simulink model "DCmotor"  (R2021a)
settings: Solver=FixedStepAuto  StartTime=0.0  StopTime=0.4  FixedStep=0.0002  RelTol=1e-3
values from neighbouring files (symbols this model uses):
  c_ss = 0.7    [Parametry_SS_motoru.m]    (also in SimRun.m = meas.c_ss + delta(5))
  J = 0.08    [Parametry_SS_motoru.m]    (also in SimRun.m = meas.J + delta(7))
  L_a = 0.8    [Parametry_SS_motoru.m]    (also in SimRun.m = meas.L_a + delta(3))
  L_b = 9.7    [Parametry_SS_motoru.m]    (also in SimRun.m = meas.L_b + delta(4))
  M_z = 0    [Parametry_SS_motoru.m]    (also in SimRun.m = meas.M_z + delta(6))
  R_a = 2.8    [Parametry_SS_motoru.m]    (also in SimRun.m = meas.R_a + delta(1))
  R_b = 8    [Parametry_SS_motoru.m]    (also in SimRun.m = meas.R_b + delta(2))
  U_a = 60.8    [Mereni.m]    (also in Optim.m = 120; Parametry_SS_motoru.m = 100; SimRun.m = U_a + delta(8))
  U_b = 27.6    [Mereni.m]    (also in Optim.m = 120; Parametry_SS_motoru.m = 120; SimRun.m = U_b + delta(9))
settings Model: Creator=liesk  LastModifiedBy=vojta
settings SolverCC: AlgebraicLoopSolver=TrustRegion
settings DebuggingCC: SFMachineParentedDataDiag=warning

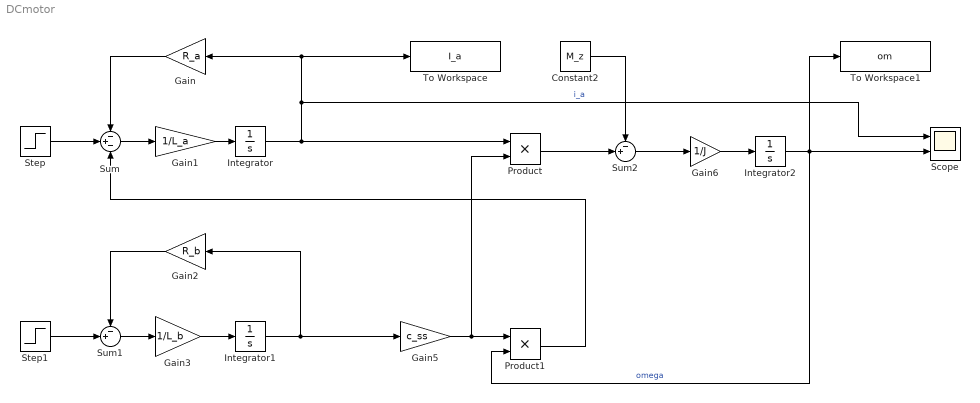
== system DCmotor ==
  Constant2 : Constant  Value=M_z
  Gain : Gain  Gain=R_a
  Gain1 : Gain  Gain=1/L_a
  Gain2 : Gain  Gain=R_b
  Gain3 : Gain  Gain=1/L_b
  Gain5 : Gain  Gain=c_ss
  Gain6 : Gain  Gain=1/J
  Integrator : Integrator
  Integrator1 : Integrator
  Integrator2 : Integrator
  Product : Product
  Product1 : Product
  Scope : Scope  NumInputPorts=2
  Step : Step  Time=0  After=U_a  SampleTime=0
  Step1 : Step  Time=0  After=U_b  SampleTime=0
  Sum : Sum  Inputs=-+-
  Sum1 : Sum  Inputs=-+|
  Sum2 : Sum  Inputs=-+|
  To Workspace : ToWorkspace  VariableName=I_a  SaveFormat=Timeseries  SampleTime=-1
  To Workspace1 : ToWorkspace  VariableName=om  SaveFormat=Timeseries  SampleTime=-1
  wires:
  Gain/1 -> Sum/1
  Sum/1 -> Gain1/1
  Gain1/1 -> Integrator/1
  Integrator/1 -> Gain/1, To Workspace/1, Scope/1, Product/1  "i_a"
  Sum1/1 -> Gain3/1
  Gain3/1 -> Integrator1/1
  Gain2/1 -> Sum1/1
  Step/1 -> Sum/2
  Step1/1 -> Sum1/2
  Product1/1 -> Sum/3
  Integrator1/1 -> Gain5/1, Gain2/1
  Gain5/1 -> Product/2, Product1/1
  Constant2/1 -> Sum2/1
  Product/1 -> Sum2/2
  Gain6/1 -> Integrator2/1
  Sum2/1 -> Gain6/1
  Integrator2/1 -> Product1/2, To Workspace1/1, Scope/2  "omega"
